simulink model "DCmotor_Speed_Ctrl"  (R2023b)
settings: Solver=FixedStepAuto  StartTime=0.0  StopTime=20  FixedStep=Ts  RelTol=1e-3
values from neighbouring files (symbols this model uses):
  J = 0.02    [DCmotor_Speed_Ctrl.m]    (also in DCmotor_Speed_Ctrl.mat)
  Kb = 0.1    [DCmotor_Speed_Ctrl.m]    (also in DCmotor_Speed_Ctrl.mat)
  Kf = 0.01    [DCmotor_Speed_Ctrl.m]    (also in DCmotor_Speed_Ctrl.mat)
  Km = 1    [DCmotor_Speed_Ctrl.m]    (also in DCmotor_Speed_Ctrl.mat)
  L = 0.5    [DCmotor_Speed_Ctrl.m]    (also in DCmotor_Speed_Ctrl.mat)
  R = 2    [DCmotor_Speed_Ctrl.m]    (also in DCmotor_Speed_Ctrl.mat)
settings Model: ExtModeTrigDuration=2  Creator=FM23  LastModifiedBy=FM23
settings OptimizationCC: EnhancedBackFolding=on  PassReuseOutputArgsAs=Individual arguments  ZeroExternalMemoryAtStartup=off  ZeroInternalMemoryAtStartup=off  MaxStackSize=64  OptimizeBlockOrder=speed  DifferentSizesBufferReuse=on  OptimizationCustomize=off  EfficientTunableParamExpr=on
settings DebuggingCC: ParameterTunabilityLossMsg=error
settings HardwareCC: ProdBitPerInt=16  ProdBitPerPointer=16  ProdBitPerSizeT=16  ProdBitPerPtrDiffT=16  ProdLargestAtomicFloat=None  ProdWordSize=8  ProdHWDeviceType=Atmel->AVR
settings SFSimCC: MATLABDynamicMemAlloc=off
settings RTWCC: Description=Embedded Coder  SystemTargetFile=ert.tlc  HardwareBoard=Arduino Mega 2560  TemplateMakefile=ert_default_tmf  Toolchain=Arduino AVR  BuildConfiguration=Faster Runs
settings CodeAppCC: ForceParamTrailComments=on  IgnoreCustomStorageClasses=off  OperatorAnnotations=on  SimulinkDataObjDesc=on  SFDataObjDesc=on  InsertBlockDesc=on
settings ERTTargetCC: SupportContinuousTime=on  SupportVariableSizeSignals=on  ExtModeTransport=3  ExtModeStaticAlloc=on  ExtModeAutomaticAllocSize=off  ExtModeStaticAllocSize=2048  ExtModeMexFile=ext_xcp  ExtModeIntrfLevel=Level2 - Open

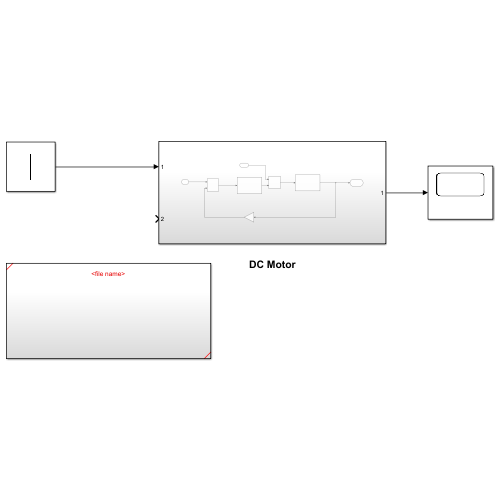
[thumbnail: Simulink's stored preview of the top-level diagram]
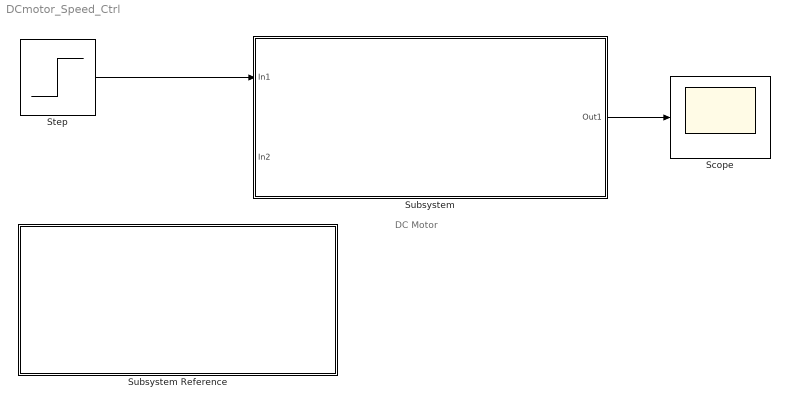
== system DCmotor_Speed_Ctrl ==
  note: DC Motor
  Scope : Scope
  Step : Step  SampleTime=0
  Subsystem : Subsystem
  Subsystem Reference : Subsystem  ReferencedSubsystem=<file name>
  wires:
  Subsystem/1(Out1) -> Scope/1
  Step/1 -> Subsystem/1(In1)

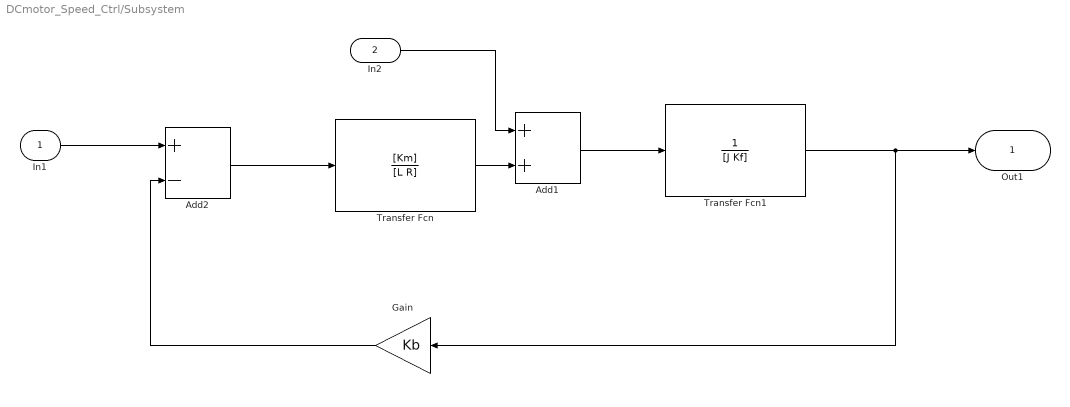
== system DCmotor_Speed_Ctrl/Subsystem ==
  In1 : Inport
  In2 : Inport  Port=2
  Add1 : Sum
  Add2 : Sum  Inputs=+-
  Gain : Gain  Gain=Kb
  Transfer Fcn : TransferFcn  Numerator=[Km]  Denominator=[L R]
  Transfer Fcn1 : TransferFcn  Denominator=[J Kf]
  Out1 : Outport
  wires:
  Transfer Fcn1/1 -> Out1/1, Gain/1
  In1/1 -> Add2/1
  Add2/1 -> Transfer Fcn/1
  Transfer Fcn/1 -> Add1/2
  In2/1 -> Add1/1
  Gain/1 -> Add2/2
  Add1/1 -> Transfer Fcn1/1

== system DCmotor_Speed_Ctrl/Subsystem Reference ==
